simulink model "SIP_lineal_y_nolineal (1)"  (R2022a)
settings: Solver=VariableStepAuto  StartTime=0.0  StopTime=3.0  MaxStep=0.01  RelTol=1e-3
values from neighbouring files (symbols this model uses):
  A = [0,0,1,0;0,0,0,1;0,a3,-a5,-a2;0,a7,-a9,-a6]    [proyecto_ss (2) (1).m]
  B = [0;0;a4;a8]    [proyecto_ss (2) (1).m]
  b2 = ng*nm*kg*kt/(Rm*rm)    (= 1.72354330709)    [proyecto_ss (2) (1).m]
  b3 = (ng*nm*kg^2*km*kt)/(Rm*rm^2)    (= 7.72356398165)    [proyecto_ss (2) (1).m]
  C = eye(4,4)    [proyecto_ss (2) (1).m]
  D = [0;0;0;0]    [proyecto_ss (2) (1).m]
undefined symbols (not defined in the file or in its folder): K
settings Model: Creator=Roberto  LastModifiedBy=Roberto

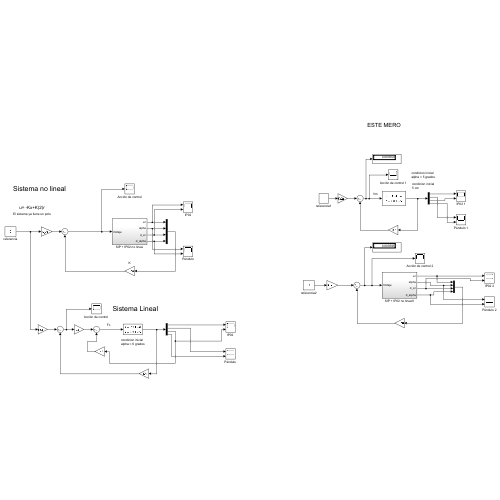
[thumbnail: Simulink's stored preview of the top-level diagram]
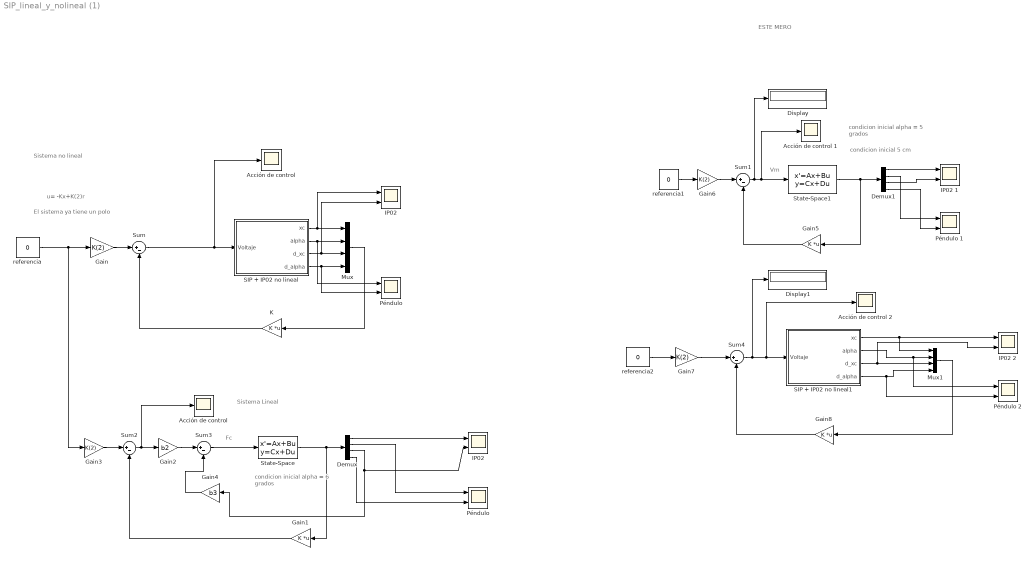
== system SIP_lineal_y_nolineal (1) ==
  note: ESTE MERO
  note: Vm
  note: Sistema Lineal
  note: Fc
  note: El sistema ya tiene un polo
  note: u= -Kx+K(2)r
  note: Sistema no lineal
  note: condicion inicial
      | alpha = 6 grados
  note: condicion inicial
      | alpha = 5 grados
  note: condicion inicial
      | 5 cm
  Acción de control : Scope
  "Acción de control " : Scope
  Acción de control 1 : Scope
  Acción de control 2 : Scope
  Demux : Demux
  Demux1 : Demux
  Display : Display
  Display1 : Display
  Gain{,3,6..7} (4 alike) : Gain  Gain=K(2)
  Gain1 : Gain  Gain=K  Multiplication=Matrix(K*u)
  Gain2 : Gain  Gain=b2
  Gain4 : Gain  Gain=b3
  Gain5 : Gain  Gain=K  Multiplication=Matrix(K*u)
  Gain8 : Gain  Gain=K  Multiplication=Matrix(K*u)
  IP02 : Scope  NumInputPorts=2
  "IP02 " : Scope  NumInputPorts=2
  IP02 1 : Scope  NumInputPorts=2
  IP02 2 : Scope  NumInputPorts=2
  K : Gain  Gain=K  Multiplication=Matrix(K*u)
  Mux : Mux
  Mux1 : Mux
  Péndulo : Scope  NumInputPorts=2
  "Péndulo " : Scope  NumInputPorts=2
  Péndulo 1 : Scope  NumInputPorts=2
  Péndulo 2 : Scope  NumInputPorts=2
  SIP + IP02 no lineal : Subsystem
  SIP + IP02 no lineal1 : Subsystem
  State-Space : StateSpace  A=A  B=B  C=C  D=[0 0 0 0]'  InitialCondition=[0.5; 0.175;0;0]
  State-Space1 : StateSpace  A=A  B=B  C=C  D=D  InitialCondition=[0.05; 0.0872;0;0]
  Sum{,1..4} (5 alike) : Sum  Inputs=|+-
  referencia : Constant  Value=0
  referencia1 : Constant  Value=0
  referencia2 : Constant  Value=0
  wires:
  SIP + IP02 no lineal/1(xc) -> IP02/1, Mux/1
  SIP + IP02 no lineal/2(alpha) -> Péndulo/1, Mux/2
  SIP + IP02 no lineal/3(d_xc) -> IP02/2, Mux/3
  SIP + IP02 no lineal/4(d_alpha) -> Péndulo/2, Mux/4
  Sum/1 -> Acción de control/1, SIP + IP02 no lineal/1(Voltaje)
  Mux/1 -> K/1
  K/1 -> Sum/2
  Gain/1 -> Sum/1
  referencia/1 -> Gain/1, Gain3/1
  Gain3/1 -> Sum2/1
  Gain1/1 -> Sum2/2
  Sum2/1 -> "Acción de control "/1, Gain2/1
  Gain2/1 -> Sum3/1
  Gain4/1 -> Sum3/2
  Sum3/1 -> State-Space/1
  Demux/3 -> Gain4/1, "IP02 "/2
  Demux/1 -> "IP02 "/1
  Demux/2 -> "Péndulo "/1
  Demux/4 -> "Péndulo "/2
  State-Space/1 -> Gain1/1, Demux/1
  Sum1/1 -> Display/1, Acción de control 1/1, State-Space1/1
  State-Space1/1 -> Gain5/1, Demux1/1
  Gain5/1 -> Sum1/2
  Demux1/1 -> IP02 1/1
  Demux1/3 -> IP02 1/2
  Demux1/2 -> Péndulo 1/1
  Demux1/4 -> Péndulo 1/2
  Gain6/1 -> Sum1/1
  referencia1/1 -> Gain6/1
  Gain7/1 -> Sum4/1
  referencia2/1 -> Gain7/1
  Sum4/1 -> Display1/1, Acción de control 2/1, SIP + IP02 no lineal1/1(Voltaje)
  SIP + IP02 no lineal1/1(xc) -> IP02 2/1, Mux1/1
  SIP + IP02 no lineal1/2(alpha) -> Péndulo 2/1, Mux1/2
  SIP + IP02 no lineal1/3(d_xc) -> IP02 2/2, Mux1/3
  SIP + IP02 no lineal1/4(d_alpha) -> Péndulo 2/2, Mux1/4
  Gain8/1 -> Sum4/2
  Mux1/1 -> Gain8/1

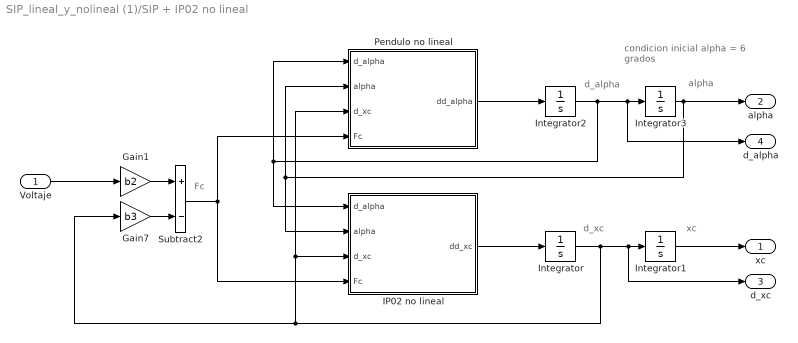
== system SIP_lineal_y_nolineal (1)/SIP + IP02 no lineal ==
  note: condicion inicial
      | alpha = 6 grados
  note: Fc
  note: xc
  note: d_xc
  note: d_alpha
  note: alpha
  Voltaje : Inport
  Gain1 : Gain  Gain=b2
  Gain7 : Gain  Gain=b3
  IP02 no lineal : MATLAB Function  TreatAsAtomicUnit=on
  Integrator : Integrator
  Integrator1 : Integrator
  Integrator2 : Integrator
  Integrator3 : Integrator  InitialCondition=0.10472
  Pendulo no lineal : MATLAB Function  TreatAsAtomicUnit=on
  Subtract2 : Sum  Inputs=+-
  xc : Outport
  alpha : Outport  Port=2
  d_xc : Outport  Port=3
  d_alpha : Outport  Port=4
  wires:
  Pendulo no lineal/1(dd_alpha) -> Integrator2/1
  Integrator/1 -> d_xc/1, Integrator1/1, Gain7/1, Pendulo no lineal/3(d_xc), IP02 no lineal/3(d_xc)
  Gain7/1 -> Subtract2/2
  Integrator3/1 -> alpha/1, IP02 no lineal/2(alpha), Pendulo no lineal/2(alpha)
  Integrator1/1 -> xc/1
  Integrator2/1 -> IP02 no lineal/1(d_alpha), Pendulo no lineal/1(d_alpha), d_alpha/1, Integrator3/1
  IP02 no lineal/1(dd_xc) -> Integrator/1
  Subtract2/1 -> Pendulo no lineal/4(Fc), IP02 no lineal/4(Fc)
  Voltaje/1 -> Gain1/1
  Gain1/1 -> Subtract2/1

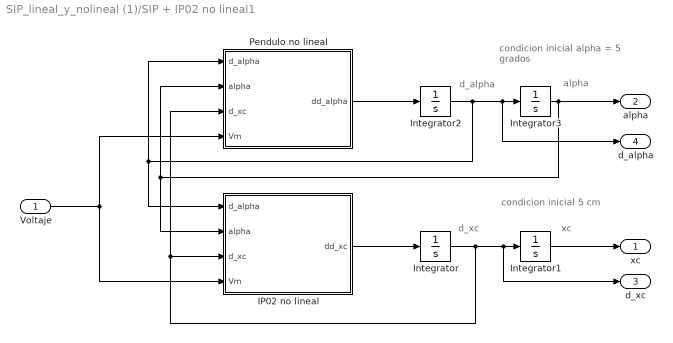
== system SIP_lineal_y_nolineal (1)/SIP + IP02 no lineal1 ==
  note: condicion inicial
      | 5 cm
  note: condicion inicial
      | alpha = 5 grados
  note: xc
  note: d_xc
  note: d_alpha
  note: alpha
  Voltaje : Inport
  IP02 no lineal : MATLAB Function  TreatAsAtomicUnit=on
  Integrator : Integrator
  Integrator1 : Integrator  InitialCondition=0.05
  Integrator2 : Integrator
  Integrator3 : Integrator  InitialCondition=0.0872
  Pendulo no lineal : MATLAB Function  TreatAsAtomicUnit=on
  xc : Outport
  alpha : Outport  Port=2
  d_xc : Outport  Port=3
  d_alpha : Outport  Port=4
  wires:
  Pendulo no lineal/1(dd_alpha) -> Integrator2/1
  Integrator/1 -> d_xc/1, Integrator1/1, Pendulo no lineal/3(d_xc), IP02 no lineal/3(d_xc)
  Integrator3/1 -> alpha/1, IP02 no lineal/2(alpha), Pendulo no lineal/2(alpha)
  Integrator1/1 -> xc/1
  Integrator2/1 -> IP02 no lineal/1(d_alpha), Pendulo no lineal/1(d_alpha), d_alpha/1, Integrator3/1
  IP02 no lineal/1(dd_xc) -> Integrator/1
  Voltaje/1 -> IP02 no lineal/4(Vm), Pendulo no lineal/4(Vm)

== matlab function SIP_lineal_y_nolineal (1)/SIP + IP02 no lineal/Pendulo no lineal ==
  data: d_alpha input; dd_alpha output; alpha input; d_xc input; Fc input
function dd_alpha = Pendulo(d_alpha,alpha,d_xc,Fc)

%--Declarar variables-- Inicio

%IP02
Jm = 3.9e-7;
Beq = 5.4;
Mc = 0.57;
nm = 1;
ng = 1;
Kg = 3.71;
Kt = 0.00767;
Km = 0.00767;
rmp = 6.35e-3;
Rm = 2.6;

%Péndulo mediano
Bp = 0.0024;
Mp = 0.127; 
Lp = 0.3365; %Largo total
lp = 0.1778; %Distancia al centro de gravedad del péndulo mediano
Ip = (1/12)*Mp*Lp^2;
g = 9.81;

%---------------------- Fin

b1 = (ng*Kg^2*Jm)/rmp^2;

dd_alpha = ((-Bp*d_alpha+Mp*g*lp*sin(alpha))*(Mc+Mp+b1)+Mp*lp*cos(alpha)*(Fc-Beq*d_xc-Mp*lp*sin(alpha)*d_alpha^2))/((Mc+Mp+b1)*(Mp*lp^2+Ip)-Mp^2*lp^2*cos(alpha)^2);

== matlab function SIP_lineal_y_nolineal (1)/SIP + IP02 no lineal/IP02 no lineal ==
  data: d_alpha input; dd_xc output; alpha input; d_xc input; Fc input
function dd_xc = IP02(d_alpha,alpha,d_xc,Fc)

%--Declarar variables-- Inicio

%IP02
Jm = 3.9e-7;
Beq = 5.4;
Mc = 0.57;
nm = 1;
ng = 1;
Kg = 3.71;
Kt = 0.00767;
Km = 0.00767;
rmp = 6.35e-3;
Rm = 2.6;

%Péndulo mediano
Bp = 0.0024;
Mp = 0.127; 
Lp = 0.3365; %Largo total
lp = 0.1778; %Distancia al centro de gravedad del péndulo mediano
Ip = (1/12)*Mp*Lp^2;
g = 9.81;

%---------------------- Fin

b1 = (ng*Kg^2*Jm)/rmp^2;

dd_xc = ((-Bp*d_alpha+Mp*g*lp*sin(alpha))*(Mp*lp*cos(alpha))+(Mp*lp^2+Ip)*(Fc-Beq*d_xc-Mp*lp*sin(alpha)*d_alpha^2))/((Mc+Mp+b1)*(Mp*lp^2+Ip)-Mp^2*lp^2*cos(alpha)^2);

== matlab function SIP_lineal_y_nolineal (1)/SIP + IP02 no lineal1/IP02 no lineal ==
  data: d_alpha input; dd_xc output; alpha input; d_xc input; Vm input
function dd_xc = IP02(d_alpha,alpha,d_xc,Vm)

%--Declarar variables-- Inicio

%IP02
Jm = 3.9e-7;
Beq = 5.4;
Mc = 0.57;
nm = 1;
ng = 1;
Kg = 3.71;
Kt = 0.00767;
Km = 0.00767;
rmp = 6.35e-3;
Rm = 2.6;

%Péndulo mediano
Bp = 0.0024;
Mp = 0.127; 
Lp = 0.3365; %Largo total
lp = 0.1778; %Distancia al centro de gravedad del péndulo mediano
Ip = (1/12)*Mp*Lp^2;
g = 9.81;

%---------------------- Fin

b1 = (ng*Kg^2*Jm)/rmp^2;
b2 = (ng*nm*Kg*Kt)/(Rm*rmp);
b3 = (ng*nm*Kg^2*Kt*Km)/(Rm*rmp^2);

dd_xc = ((-Bp*d_alpha+Mp*g*lp*sin(alpha))*(Mp*lp*cos(alpha))+(Mp*lp^2+Ip)*(b2*Vm-b3*d_xc-Beq*d_xc-Mp*lp*sin(alpha)*d_alpha^2))/((Mc+Mp+b1)*(Mp*lp^2+Ip)-Mp^2*lp^2*cos(alpha)^2);

== matlab function SIP_lineal_y_nolineal (1)/SIP + IP02 no lineal1/Pendulo no lineal ==
  data: d_alpha input; dd_alpha output; alpha input; d_xc input; Vm input
function dd_alpha = Pendulo(d_alpha,alpha,d_xc,Vm)

%--Declarar variables-- Inicio

%IP02
Jm = 3.9e-7;
Beq = 5.4;
Mc = 0.57;
nm = 1;
ng = 1;
Kg = 3.71;
Kt = 0.00767;
Km = 0.00767;
rmp = 6.35e-3;
Rm = 2.6;

%Péndulo mediano
Bp = 0.0024;
Mp = 0.127; 
Lp = 0.3365; %Largo total
lp = 0.1778; %Distancia al centro de gravedad del péndulo mediano
Ip = (1/12)*Mp*Lp^2;
g = 9.81;

%---------------------- Fin

b1 = (ng*Kg^2*Jm)/rmp^2;
b2 = (ng*nm*Kg*Kt)/(Rm*rmp);
b3 = (ng*nm*Kg^2*Kt*Km)/(Rm*rmp^2);

dd_alpha = ((-Bp*d_alpha+Mp*g*lp*sin(alpha))*(Mc+Mp+b1)+Mp*lp*cos(alpha)*(b2*Vm-b3*d_xc-Beq*d_xc-Mp*lp*sin(alpha)*d_alpha^2))/((Mc+Mp+b1)*(Mp*lp^2+Ip)-Mp^2*lp^2*cos(alpha)^2);
